simulink model "Strecke"  (R2021a)
settings: Solver=ode23s  StartTime=0.0  StopTime=5  FixedStep=0.0001  MaxStep=1e-3  RelTol=1e-3  EnableMultiTasking=on
values from neighbouring files (symbols this model uses):
  friction_gain = 5.55028e-07    [params_m.m]    (also in strecke_params_m.m = 6e-07)
  J = Jk    (= 7e-07)    [params_m.m]    (also in strecke_params_m.m = 1e-06)
  km = 14.8e-3    (= 0.0148)    [params_m.m]    (also in strecke_params_m.m)
  L = 2e-3    (= 0.002)    [params_m.m]    (also in strecke_params_m.m)
  omega_AW = 0    [params_m.m]    (also in strecke_params_m.m)
  phi_AW = 0 * pi / 180    (= 0)    [params_m.m]    (also in strecke_params_m.m)
  R = 11.9    [params_m.m]    (also in strecke_params_m.m)
  R_Lampe = 12.4    [params_m.m]    (also in strecke_params_m.m)
  R_shunt = 1.0    (= 1)    [params_m.m]    (also in strecke_params_m.m)
settings Model: Creator=Walter Lindermeir  LastModifiedBy=maowit00
settings SolverCC: AlgebraicLoopSolver=TrustRegion
settings DataIOCC: LimitDataPoints=on  SaveFormat=Array  ReturnWorkspaceOutputs=off
settings OptimizationCC: ExpressionDepthLimit=2147483647  EfficientFloat2IntCast=on  LifeSpan=inf
settings DebuggingCC: SaveWithParameterizedLinksMsg=none  SignalResolutionControl=TryResolveAllWithWarning  SolverPrmCheckMsg=warning  AllowSymbolicDim=off  StateNameClashWarn=warning  StrictBusMsg=ErrorOnBusTreatedAsVector  SFUnexpectedBacktrackingDiag=warning  SFNoUnconditionalDefaultTransitionDiag=warning  SFExecutionAtInitializationDiag=none  SFMachineParentedDataDiag=warning  ArithmeticOperatorsInVariantConditions=warning
settings HardwareCC: ProdBitPerPointer=32  ProdBitPerSizeT=32  ProdBitPerPtrDiffT=32  ProdLargestAtomicFloat=None  ProdIntDivRoundTo=Undefined  ProdEndianess=Unspecified  ProdWordSize=32  ProdHWDeviceType=32-bit Generic
settings ModelReferenceCC: PropagateSignalLabelsOutOfModel=off
settings SFSimCC: SimUseLocalCustomCode=off  CustomCodeUndefinedFunction=UseInterfaceOnly
settings RTWCC: RTWUseLocalCustomCode=off
settings CodeAppCC: StateflowObjectComments=on
settings GRTTargetCC: TargetFcnLib=ansi_tfl_tmw.mat  TargetLangStandard=C89/C90 (ANSI)  CombineOutputUpdateFcns=off  GRTInterface=on
settings ConfigComp: CovMetricSettings=dw  CovSaveCumulativeToWorkspaceVar=on  CovSaveSingleToWorkspaceVar=on  CovExternalEMLEnable=off

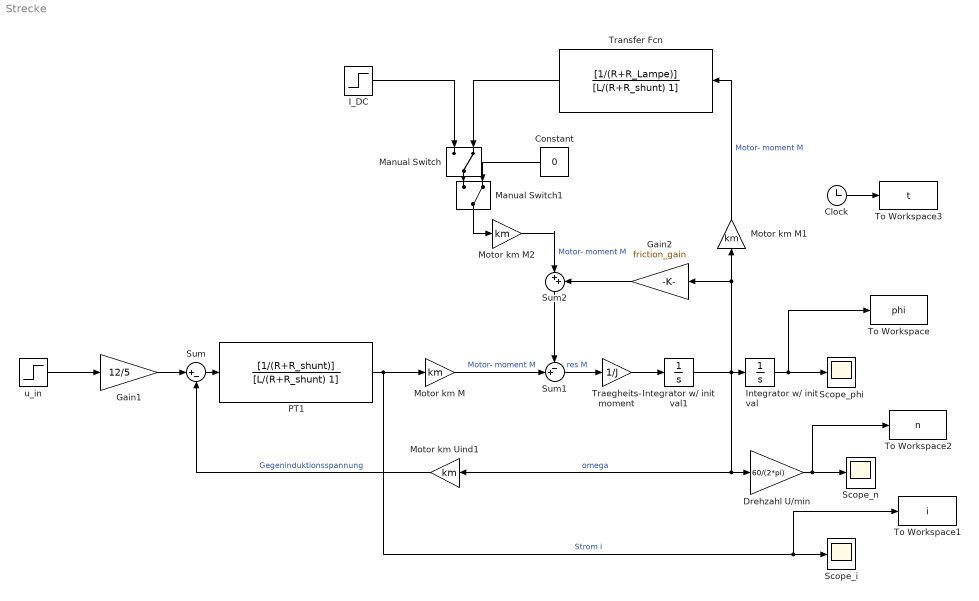
== system Strecke ==
  Clock : Clock
  Constant : Constant  Value=0
  Drehzahl U/min : Gain  Gain=60/(2*pi)
  Gain1 : Gain  Gain=12/5
  Gain2 : Gain  Gain=friction_gain
  I_DC : Step  Time=3  After=0.2  SampleTime=0
  Integrator w/ init val : Integrator  InitialCondition=phi_AW
  Integrator w/ init val1 : Integrator  InitialCondition=omega_AW
  Manual Switch : ManualSwitch  CurrentSetting=0
  Manual Switch1 : ManualSwitch  CurrentSetting=0
  Motor km M : Gain  Gain=km
  Motor km M1 : Gain  Gain=km
  Motor km M2 : Gain  Gain=km
  Motor km Uind1 : Gain  Gain=km
  PT1 : TransferFcn  Numerator=[1/(R+R_shunt)]  Denominator=[L/(R+R_shunt) 1]
  Scope_i : Scope
  Scope_n : Scope
  Scope_phi : Scope
  Sum : Sum  Inputs=|+-
  Sum1 : Sum  Inputs=-+|
  Sum2 : Sum  Inputs=|++
  To Workspace : ToWorkspace  VariableName=phi  SampleTime=-1
      settings: Save2DSignal=2-D array (concatenate along first dimension)
  To Workspace1 : ToWorkspace  VariableName=i  SampleTime=-1
      settings: Save2DSignal=2-D array (concatenate along first dimension)
  To Workspace2 : ToWorkspace  VariableName=n  SampleTime=-1
      settings: Save2DSignal=2-D array (concatenate along first dimension)
  To Workspace3 : ToWorkspace  VariableName=t  SampleTime=-1
      settings: Save2DSignal=2-D array (concatenate along first dimension)
  Traegheits- moment : Gain  Gain=1/J
  Transfer Fcn : TransferFcn  Numerator=[1/(R+R_Lampe)]  Denominator=[L/(R+R_shunt) 1]
  u_in : Step  After=4  SampleTime=0
  wires:
  PT1/1 -> Scope_i/1, To Workspace1/1, Motor km M/1  "Strom i"
  Motor km M/1 -> Sum1/2  "Motor- moment M"
  Integrator w/ init val1/1 -> Integrator w/ init val/1, Motor km M1/1, Gain2/1, Drehzahl U/min/1, Motor km Uind1/1  "omega"
  Integrator w/ init val/1 -> Scope_phi/1, To Workspace/1
  Gain1/1 -> Sum/1
  Sum1/1 -> Traegheits- moment/1  "res M"
  Motor km Uind1/1 -> Sum/2  "Gegeninduktionsspannung"
  u_in/1 -> Gain1/1
  Sum/1 -> PT1/1
  Traegheits- moment/1 -> Integrator w/ init val1/1
  Drehzahl U/min/1 -> Scope_n/1, To Workspace2/1
  Clock/1 -> To Workspace3/1
  Sum2/1 -> Sum1/1
  Gain2/1 -> Sum2/2
  Motor km M1/1 -> Transfer Fcn/1  "Motor- moment M"
  Manual Switch/1 -> Manual Switch1/1
  Constant/1 -> Manual Switch1/2
  Manual Switch1/1 -> Motor km M2/1
  Motor km M2/1 -> Sum2/1  "Motor- moment M"
  Transfer Fcn/1 -> Manual Switch/2
  I_DC/1 -> Manual Switch/1
